simulink model "anc1"  (Simulink 4.00)
settings: Solver=ode45  StartTime=0.0  StopTime=1000000  RelTol=1e-3
libraries: dspsrcs3 x2, dspsnks3 x1
settings Model: LastModifiedBy=admin

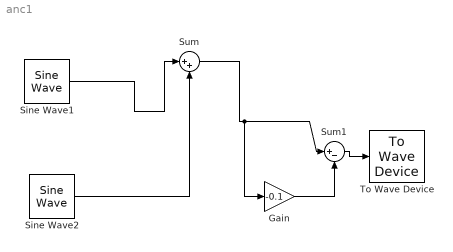
== system anc1 ==
  Gain : Gain  Gain=-0.1  Multiplication=Element-wise(K.*u)  SaturateOnIntegerOverflow=on
  Sine Wave1 : dspsrcs3/Sine Wave  Amplitude=1  Frequency=15  Phase=0  SampleMode=Discrete  OutComplex=Real  CompMethod=Trigonometric Fcn  TableSize=Speed  SampleTime=1/1000  SamplesPerFrame=1  ResetState=Restart at time zero
  Sine Wave2 : dspsrcs3/Sine Wave  Amplitude=1  Frequency=150  Phase=0  SampleMode=Discrete  OutComplex=Real  CompMethod=Trigonometric Fcn  TableSize=Speed  SampleTime=1/1000  SamplesPerFrame=1  ResetState=Restart at time zero
  Sum : Sum  Inputs=|++  SaturateOnIntegerOverflow=on
  Sum1 : Sum  Inputs=|+-  SaturateOnIntegerOverflow=on
  To Wave Device : dspsnks3/To Wave Device  bufDuration=2  initDelay=0.1  useDefaultDevice=on  userDeviceID=1
  wires:
  Sine Wave1/1 -> Sum/1
  Sine Wave2/1 -> Sum/2
  Sum/1 -> Gain/1, Sum1/1
  Gain/1 -> Sum1/2
  Sum1/1 -> To Wave Device/1
